simulink model "test_case_old"  (R2014a)
settings: Solver=ode3  StartTime=0.0  StopTime=1*24*3600  FixedStep=1  RelTol=1e-3
libraries: caselibrary x1
settings Model: Creator=avenger  LastModifiedBy=avenger

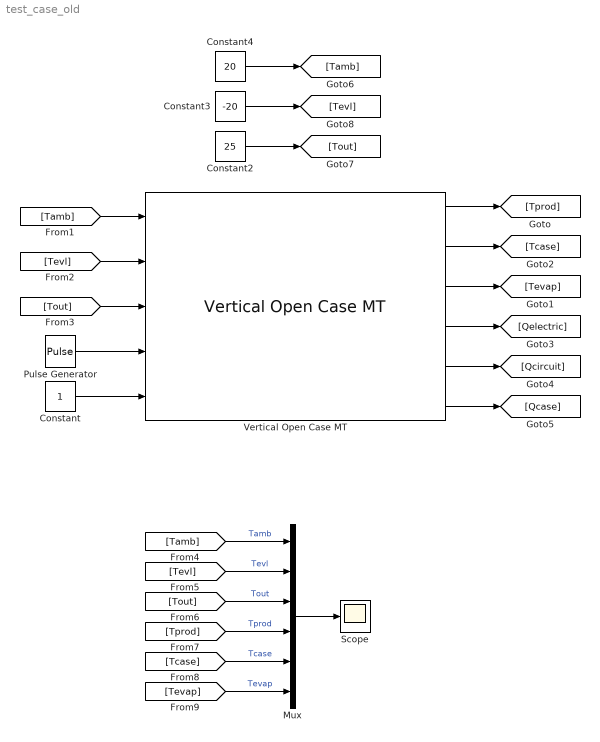
== system test_case_old ==
  Constant : Constant
  Constant2 : Constant  Value=25
  Constant3 : Constant  Value=-20
  Constant4 : Constant  Value=20
  Mux : Mux  Inputs=6
  Pulse Generator : DiscretePulseGenerator  PulseType=Time based  Period=24*3600  PulseWidth=100*1/24  PhaseDelay=12*3600
  Scope : Scope
      settings: ShowLegends=on  YMin=-22.5  YMax=32.5
  Vertical Open Case MT : caselibrary/Vertical Open Case MT
  wires:
  Vertical Open Case MT/1 -> [Tprod]
  Vertical Open Case MT/2 -> [Tcase]
  Vertical Open Case MT/3 -> [Tevap]
  Vertical Open Case MT/4 -> [Qelectric]
  Vertical Open Case MT/5 -> [Qcircuit]
  Vertical Open Case MT/6 -> [Qcase]
  Pulse Generator/1 -> Vertical Open Case MT/4
  [Tevl] -> Vertical Open Case MT/2
  [Tout] -> Vertical Open Case MT/3
  Constant/1 -> Vertical Open Case MT/5
  [Tamb] -> Vertical Open Case MT/1
  Mux/1 -> Scope/1
  [Tevl] -> Mux/2  "Tevl"
  [Tout] -> Mux/3  "Tout"
  [Tamb] -> Mux/1  "Tamb"
  [Tcase] -> Mux/5  "Tcase"
  [Tevap] -> Mux/6  "Tevap"
  [Tprod] -> Mux/4  "Tprod"
  Constant4/1 -> [Tamb]
  Constant3/1 -> [Tevl]
  Constant2/1 -> [Tout]
